simulink model "mod1"  (R2019a)
settings: Solver=VariableStepAuto  StartTime=0.0  StopTime=10.0  RelTol=1e-3
settings Model: Creator=step_oda  LastModifiedBy=bomjz
settings DataIOCC: ReturnWorkspaceOutputs=off
settings DebuggingCC: ArithmeticOperatorsInVariantConditions=warning
settings SFSimCC: SimUseLocalCustomCode=off
settings RTWCC: RTWUseLocalCustomCode=off
settings CodeAppCC: StateflowObjectComments=on

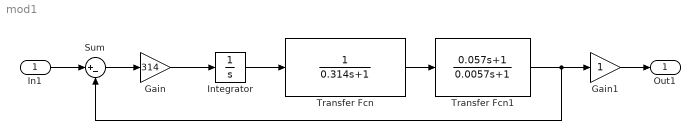
== system mod1 ==
  In1 : Inport
  Gain : Gain  Gain=314
  Gain1 : Gain
  Integrator : Integrator
  Sum : Sum  Inputs=|+-
  Transfer Fcn : TransferFcn  Denominator=[0.314 1]
  Transfer Fcn1 : TransferFcn  Numerator=[0.057 1]  Denominator=[0.0057 1]
  Out1 : Outport
  wires:
  Gain/1 -> Integrator/1
  Integrator/1 -> Transfer Fcn/1
  Sum/1 -> Gain/1
  In1/1 -> Sum/1
  Transfer Fcn/1 -> Transfer Fcn1/1
  Gain1/1 -> Out1/1
  Transfer Fcn1/1 -> Sum/2, Gain1/1
